simulink model "GMP_STD_CLLLC_MODEL"  (R2024b)
settings: Solver=FixedStepDiscrete  StartTime=0.0  StopTime=0.02  FixedStep=2e-8  RelTol=1e-3
PostLoadFcn:
  | gmp_model_file=get_param(bdroot,'FileName'); if isempty(gmp_model_file), error('GMP:SDPE:ModelPath','The model must be saved before SDPE initialization.'); end; gmp_model_dir=fileparts(gmp_model_file); run(fullfile(gmp_model_dir,'sdpe_mgr','ctrl_settings_matlab_init.m')); gmp_matlab_release=matlabRelease; gmp_repo_root=fullfile(gmp_model_dir,'..','..','..','..','..'); addpath(fullfile(gmp_repo_root,'slib','install_path',gmp_matlab_release.Release,'src')); clear gmp_model_file gmp_model_dir gmp_matlab_release gmp_repo_root;
InitFcn:
  | gmp_model_file=get_param(bdroot,'FileName'); if isempty(gmp_model_file), error('GMP:SDPE:ModelPath','The model must be saved before SDPE initialization.'); end; gmp_model_dir=fileparts(gmp_model_file); run(fullfile(gmp_model_dir,'sdpe_mgr','ctrl_settings_matlab_init.m')); gmp_matlab_release=matlabRelease; gmp_repo_root=fullfile(gmp_model_dir,'..','..','..','..','..'); addpath(fullfile(gmp_repo_root,'slib','install_path',gmp_matlab_release.Release,'src')); clear gmp_model_file gmp_model_dir gmp_matlab_release gmp_repo_root;
libraries: spsSeriesRLCBranchLib x4, spsCurrentMeasurementLib x3, spsUniversalBridgeLib x2, spsVoltageMeasurementLib x2, gmp_sil_core_pack x1, spsLinearTransformerLib x1, spsDCVoltageSourceLib x1, spsGroundLib x1, spspowerguiLib x1
settings Model: Creator=javnson  LastModifiedBy=javnson

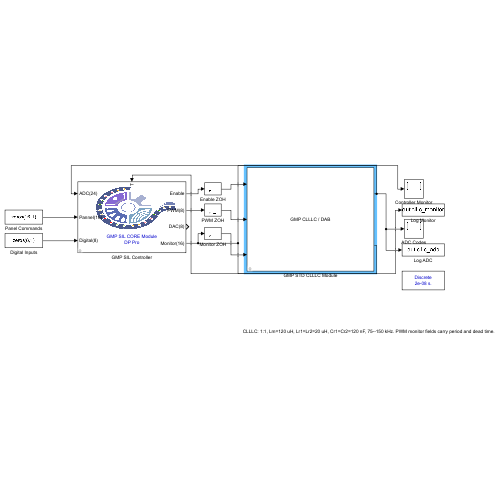
[thumbnail: Simulink's stored preview of the top-level diagram]
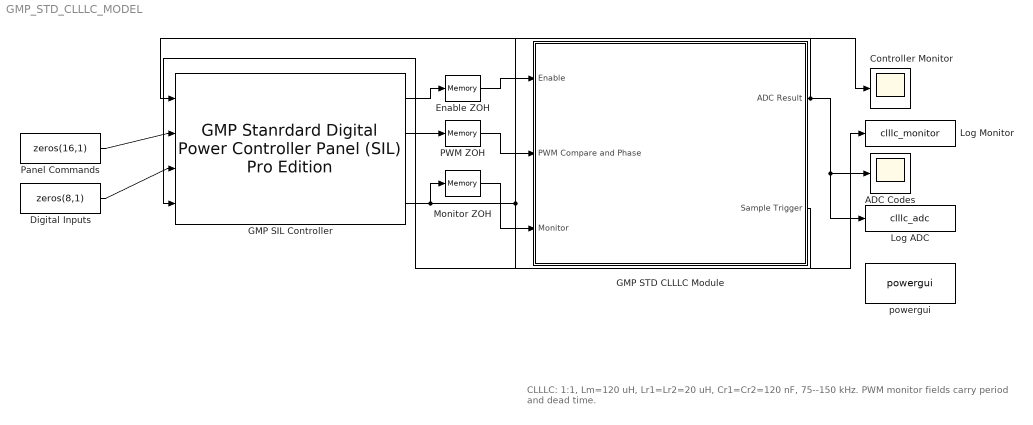
== system GMP_STD_CLLLC_MODEL ==
  note: CLLLC: 1:1, Lm=120 uH, Lr1=Lr2=20 uH, Cr1=Cr2=120 nF, 75--150 kHz. PWM monitor fields carry period and dead time.
  ADC Codes : Scope
  Controller Monitor : Scope
  Digital Inputs : Constant  Value=zeros(8,1)
  Enable ZOH : Memory
  GMP SIL Controller : gmp_sil_core_pack/GMP Stanrdard Digital Power Controller Panel (SIL) Pro Edition
      settings: SourceProductName=GMP SIL Core Utilities
  GMP STD CLLLC Module : Subsystem
      mask DialogControl TankGroup Prompt: Resonant Tank (SDPE synchronized)
      mask DialogControl SensorGroup Prompt: ADC Sensors
      mask DialogControl PwmGroup Prompt: PWM and Sampling
      mask Display: disp('GMP CLLLC / DAB')
  Log ADC : ToWorkspace  VariableName=clllc_adc  SaveFormat=Timeseries  SampleTime=-1
  Log Monitor : ToWorkspace  VariableName=clllc_monitor  SaveFormat=Timeseries  SampleTime=-1
  Monitor ZOH : Memory  InitialCondition=zeros(16,1)
  PWM ZOH : Memory  InitialCondition=zeros(8,1)
  Panel Commands : Constant  Value=zeros(16,1)
  powergui : spspowerguiLib/powergui  Priority=1  SimulationMode=Discrete  SampleTime=2e-8  frequency=60  Iterations=50  frequencyindice=60  Pbase=100e6  ErrMax=1e-4  UnitsV=kV  UnitsW=MW  buscounter=0  FunctionMessages=off  echomessages=off  EnableUseOfTLC=off  CurrentSourceSwitches=off  DisableSnubberDevices=off  DisableRonSwitches=off  DisableVfSwitches=off  DisplayEquations=off  AutomaticDiscreteSolvers=off  SolverType=Tustin/Backward Euler (TBE)  Interpol=off  ExternalGateDelay=off  methode=off  Ts=100  x0status=blocks  SPID=on  SwTol=0  HookPort=off  NonlinearTolerance=1e-4  nMaxIteration=100  ContinueOnMaxIteration=off  RestoreLinks=warning  ResistiveCurrentMeasurement=off  Frange=[0:2:500]  Ylog=off  Xlog=on  ShowGrid=off  save=off  variable=ZData  structure=0  ZoomFFT=off  StartTime=0.0  cycles=1  DisplayStyle=1  fundamental=60  FreqAxis=off  MaxFrequency=1000  frequencyindicesteady=1  RmsSteady=1  display=off
  wires:
  GMP STD CLLLC Module/1(ADC Result) -> ADC Codes/1, Log ADC/1, GMP SIL Controller/1
  Panel Commands/1 -> GMP SIL Controller/2
  Digital Inputs/1 -> GMP SIL Controller/3
  GMP STD CLLLC Module/2(Sample Trigger) -> GMP SIL Controller/4
  GMP SIL Controller/1 -> Enable ZOH/1
  GMP SIL Controller/2 -> PWM ZOH/1
  GMP SIL Controller/4 -> Controller Monitor/1, Log Monitor/1, Monitor ZOH/1
  Enable ZOH/1 -> GMP STD CLLLC Module/1(Enable)
  PWM ZOH/1 -> GMP STD CLLLC Module/2(PWM Compare and Phase)
  Monitor ZOH/1 -> GMP STD CLLLC Module/3(Monitor)

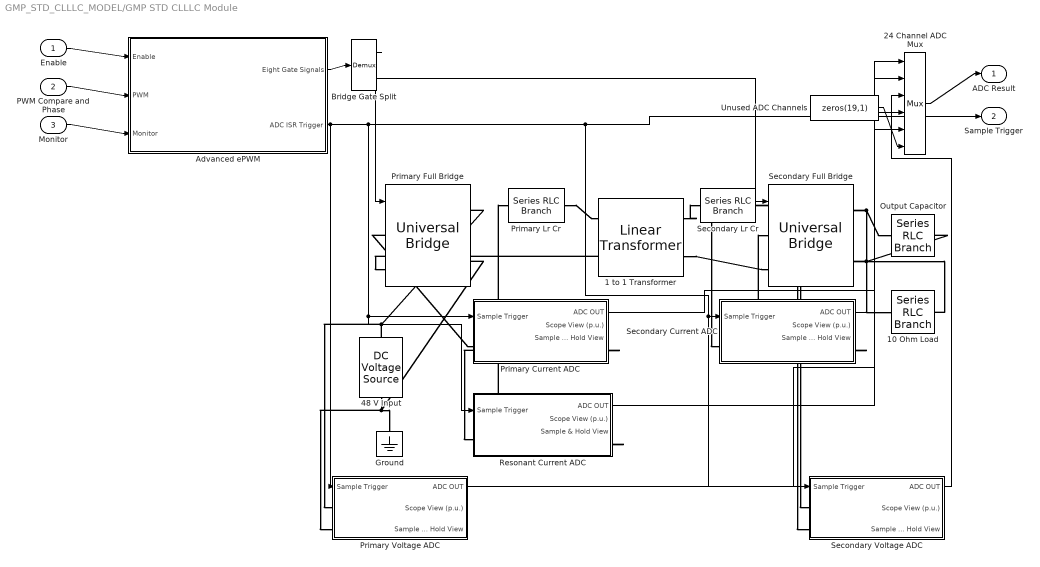
== system GMP_STD_CLLLC_MODEL/GMP STD CLLLC Module ==
  Enable : Inport
  PWM Compare and Phase : Inport  Port=2
  Monitor : Inport  Port=3
  1 to 1 Transformer : spsLinearTransformerLib/Linear Transformer  UNITS=SI  NominalPower=[1000 100e3]  winding1=[48 0.01 1e-9]  winding2=[48 0.01 1e-9]  ThreeWindings=off  winding3=[3.15e+05 0.7938 0.084225]  RmLm=[1e6 120e-6]  Measurements=None  DataType=on
  10 Ohm Load : spsSeriesRLCBranchLib/Series RLC Branch  LConnTagsString=__new0  RConnTagsString=__new0  BranchType=R  Resistance=10  Inductance=1e-3  SetiL0=off  InitialCurrent=0  Capacitance=1e-6  Setx0=off  InitialVoltage=0  Measurements=None
  24 Channel ADC Mux : Mux  Inputs=6
  48 V Input : spsDCVoltageSourceLib/DC Voltage Source  Amplitude=48  Measurements=None
  Advanced ePWM : Subsystem  mask{TimerClockHz=100e6, NominalPeriodTicks=1000, DeadtimeSeconds=200e-9, AdcCyclesPerIsr=2}
      mask prompts: TimerClockHz "Timer clock (Hz)"; NominalPeriodTicks "Nominal period ticks"; DeadtimeSeconds "Nominal dead time (s)"; AdcCyclesPerIsr "PWM cycles per ADC/ISR"
      mask DialogControl Timebase Prompt: Timebase and Frequency
      mask DialogControl Deadband Prompt: Complementary Dead Band
      mask DialogControl Sampling Prompt: ADC / ISR Trigger
      mask Display: disp('Advanced ePWM\nF/Phase/Duty/Deadtime')
  Bridge Gate Split : Demux  Outputs=[4 4]
  Ground : spsGroundLib/Ground  LConnTagsString=a
  Output Capacitor : spsSeriesRLCBranchLib/Series RLC Branch  LConnTagsString=__new0  RConnTagsString=__new0  BranchType=C  Resistance=1  Inductance=1e-3  SetiL0=off  InitialCurrent=0  Capacitance=440e-6  Setx0=off  InitialVoltage=0  Measurements=None
  Primary Current ADC : Subsystem  mask{ADC_GAIN=0.15, ADC_BIT=12, ADC_REFERENCE=3.3, ADC_BIAS=1.65, ADC_INIT=2048}
      mask DialogControl DescGroupVar Prompt: Current Sample ADC Model 1
      mask DialogControl DescTextVar Prompt: This is a ideal Current Measurement Module. This module enable a bias and a gain, and finally output a ADC result.
      mask DialogControl Control8 Prompt: ADC(p.u.) = (real_current * ADC_GAIN + ADC_BIAS)/ADC_REFERENCE
      mask DialogControl Control9 Prompt: GMP CTL Simulink Utilities: virtual peripherals
      mask DialogControl ParameterGroupVar Prompt: 参数
      mask DialogControl Control7 Prompt: ADC Current Gain (Scale Factor):
      mask DialogControl Control2 Prompt: ADC resolution:
      mask DialogControl Control4 Prompt: ADC reference Current(A), ADC full scale current (when gain = 1)
      mask DialogControl Control5 Prompt: ADC Bias Current(A)
      mask DialogControl Control6 Prompt: ADC initial Current Output(A)
  Primary Full Bridge : spsUniversalBridgeLib/Universal Bridge  Arms=2  SnubberResistance=1e6  SnubberCapacitance=inf  Device=MOSFET / Diodes  Ron=0.01  Lon=0  ForwardVoltages="[  0  0  ]"  ForwardVoltage=0  GTOparameters=[ 10e-6 , 20e-6 ]  IGBTparameters=[ 1e-6 , 2e-6 ]  Measurements=None  Measurements_2=None  converterType=Rectifier
  Primary Lr Cr : spsSeriesRLCBranchLib/Series RLC Branch  LConnTagsString=__new0  RConnTagsString=__new0  BranchType=RLC  Resistance=0.05  Inductance=20e-6  SetiL0=off  InitialCurrent=0  Capacitance=120e-9  Setx0=off  InitialVoltage=0  Measurements=None
  Primary Voltage ADC : Subsystem  mask{ADC_GAIN=0.02705, ADC_BIT=12, ADC_REFERENCE=3.3, ADC_BIAS=0, ADC_INIT=0}
      mask DialogControl DescGroupVar Prompt: Voltage Sample ADC Model
      mask DialogControl DescTextVar Prompt: This is a ideal Voltage Measurement Module.
      mask DialogControl Control2 Prompt: ADC(p.u.) = (real_voltage * ADC_GAIN + ADC_BIAS)/ADC_REFERENCE
      mask DialogControl Control9 Prompt: GMP CTL Simulink Utilities: virtual peripherals
      mask DialogControl ParameterGroupVar Prompt: Parameters:
      mask DialogControl Control4 Prompt: ADC Voltage Gain (Scale Factor):
      mask DialogControl Control5 Prompt: ADC resolution:
      mask DialogControl Control6 Prompt: ADC reference Voltage(V)
      mask DialogControl Control8 Prompt: ADC Bias Voltage(V)
      mask DialogControl Control7 Prompt: ADC Initial Voltage Output (V):
  Resonant Current ADC : Subsystem  mask{ADC_GAIN=0.15, ADC_BIT=12, ADC_REFERENCE=3.3, ADC_BIAS=1.65, ADC_INIT=2048}
      mask DialogControl DescGroupVar Prompt: Current Sample ADC Model 1
      mask DialogControl DescTextVar Prompt: This is a ideal Current Measurement Module. This module enable a bias and a gain, and finally output a ADC result.
      mask DialogControl Control8 Prompt: ADC(p.u.) = (real_current * ADC_GAIN + ADC_BIAS)/ADC_REFERENCE
      mask DialogControl Control9 Prompt: GMP CTL Simulink Utilities: virtual peripherals
      mask DialogControl ParameterGroupVar Prompt: 参数
      mask DialogControl Control7 Prompt: ADC Current Gain (Scale Factor):
      mask DialogControl Control2 Prompt: ADC resolution:
      mask DialogControl Control4 Prompt: ADC reference Current(A), ADC full scale current (when gain = 1)
      mask DialogControl Control5 Prompt: ADC Bias Current(A)
      mask DialogControl Control6 Prompt: ADC initial Current Output(A)
  Secondary Current ADC : Subsystem  mask{ADC_GAIN=0.15, ADC_BIT=12, ADC_REFERENCE=3.3, ADC_BIAS=1.65, ADC_INIT=2048}
      mask DialogControl DescGroupVar Prompt: Current Sample ADC Model 1
      mask DialogControl DescTextVar Prompt: This is a ideal Current Measurement Module. This module enable a bias and a gain, and finally output a ADC result.
      mask DialogControl Control8 Prompt: ADC(p.u.) = (real_current * ADC_GAIN + ADC_BIAS)/ADC_REFERENCE
      mask DialogControl Control9 Prompt: GMP CTL Simulink Utilities: virtual peripherals
      mask DialogControl ParameterGroupVar Prompt: 参数
      mask DialogControl Control7 Prompt: ADC Current Gain (Scale Factor):
      mask DialogControl Control2 Prompt: ADC resolution:
      mask DialogControl Control4 Prompt: ADC reference Current(A), ADC full scale current (when gain = 1)
      mask DialogControl Control5 Prompt: ADC Bias Current(A)
      mask DialogControl Control6 Prompt: ADC initial Current Output(A)
  Secondary Full Bridge : spsUniversalBridgeLib/Universal Bridge  Arms=2  SnubberResistance=1e6  SnubberCapacitance=inf  Device=MOSFET / Diodes  Ron=0.01  Lon=0  ForwardVoltages="[  0  0  ]"  ForwardVoltage=0  GTOparameters=[ 10e-6 , 20e-6 ]  IGBTparameters=[ 1e-6 , 2e-6 ]  Measurements=None  Measurements_2=None  converterType=Rectifier
  Secondary Lr Cr : spsSeriesRLCBranchLib/Series RLC Branch  LConnTagsString=__new0  RConnTagsString=__new0  BranchType=RLC  Resistance=0.05  Inductance=20e-6  SetiL0=off  InitialCurrent=0  Capacitance=120e-9  Setx0=off  InitialVoltage=0  Measurements=None
  Secondary Voltage ADC : Subsystem  mask{ADC_GAIN=0.02705, ADC_BIT=12, ADC_REFERENCE=3.3, ADC_BIAS=0, ADC_INIT=0}
      mask DialogControl DescGroupVar Prompt: Voltage Sample ADC Model
      mask DialogControl DescTextVar Prompt: This is a ideal Voltage Measurement Module.
      mask DialogControl Control2 Prompt: ADC(p.u.) = (real_voltage * ADC_GAIN + ADC_BIAS)/ADC_REFERENCE
      mask DialogControl Control9 Prompt: GMP CTL Simulink Utilities: virtual peripherals
      mask DialogControl ParameterGroupVar Prompt: Parameters:
      mask DialogControl Control4 Prompt: ADC Voltage Gain (Scale Factor):
      mask DialogControl Control5 Prompt: ADC resolution:
      mask DialogControl Control6 Prompt: ADC reference Voltage(V)
      mask DialogControl Control8 Prompt: ADC Bias Voltage(V)
      mask DialogControl Control7 Prompt: ADC Initial Voltage Output (V):
  Unused ADC Channels : Constant  Value=zeros(19,1)  OutDataTypeStr=uint32
  ADC Result : Outport
  Sample Trigger : Outport  Port=2
  wires:
  Enable/1 -> Advanced ePWM/1(Enable)
  PWM Compare and Phase/1 -> Advanced ePWM/2(PWM)
  Monitor/1 -> Advanced ePWM/3(Monitor)
  Advanced ePWM/2(ADC ISR Trigger) -> Primary Current ADC/1(Sample Trigger), Resonant Current ADC/1(Sample Trigger), Secondary Voltage ADC/1(Sample Trigger), Secondary Current ADC/1(Sample Trigger), Sample Trigger/1, Primary Voltage ADC/1(Sample Trigger)
  Advanced ePWM/1(Eight Gate Signals) -> Bridge Gate Split/1
  Bridge Gate Split/1 -> Primary Full Bridge/1
  Bridge Gate Split/2 -> Secondary Full Bridge/1
  Primary Voltage ADC/1(ADC OUT) -> 24 Channel ADC Mux/1
  Primary Current ADC/1(ADC OUT) -> 24 Channel ADC Mux/2
  Secondary Voltage ADC/1(ADC OUT) -> 24 Channel ADC Mux/3
  Secondary Current ADC/1(ADC OUT) -> 24 Channel ADC Mux/4
  Resonant Current ADC/1(ADC OUT) -> 24 Channel ADC Mux/5
  Unused ADC Channels/1 -> 24 Channel ADC Mux/6
  24 Channel ADC Mux/1 -> ADC Result/1
  connections:
  Primary Full Bridge/RConn1 -- 48 V Input/RConn1 -- Primary Voltage ADC/LConn1
  Primary Full Bridge/RConn2 -- 48 V Input/LConn1 -- Ground/LConn1 -- Primary Voltage ADC/LConn2
  Primary Full Bridge/LConn1 -- Primary Current ADC/LConn1
  Primary Current ADC/RConn1 -- Resonant Current ADC/LConn1
  Resonant Current ADC/RConn1 -- Primary Lr Cr/LConn1
  Primary Lr Cr/RConn1 -- 1 to 1 Transformer/LConn1
  1 to 1 Transformer/LConn2 -- Primary Full Bridge/LConn2
  1 to 1 Transformer/RConn1 -- Secondary Lr Cr/LConn1
  Secondary Lr Cr/RConn1 -- Secondary Current ADC/LConn1
  Secondary Current ADC/RConn1 -- Secondary Full Bridge/LConn1
  1 to 1 Transformer/RConn2 -- Secondary Full Bridge/LConn2
  Output Capacitor/LConn1 -- Secondary Full Bridge/RConn1 -- 10 Ohm Load/LConn1 -- Secondary Voltage ADC/LConn1
  Output Capacitor/RConn1 -- Secondary Full Bridge/RConn2 -- 10 Ohm Load/RConn1 -- Secondary Voltage ADC/LConn2

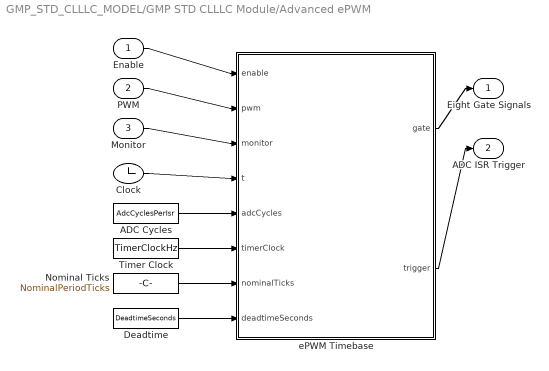
== system GMP_STD_CLLLC_MODEL/GMP STD CLLLC Module/Advanced ePWM ==
  Enable : Inport
  PWM : Inport  Port=2
  Monitor : Inport  Port=3
  ADC Cycles : Constant  Value=AdcCyclesPerIsr
  Clock : Clock
  Deadtime : Constant  Value=DeadtimeSeconds
  Nominal Ticks : Constant  Value=NominalPeriodTicks
  Timer Clock : Constant  Value=TimerClockHz
  ePWM Timebase : MATLAB Function  TreatAsAtomicUnit=on
  Eight Gate Signals : Outport
  ADC ISR Trigger : Outport  Port=2
  wires:
  Enable/1 -> ePWM Timebase/1(enable)
  PWM/1 -> ePWM Timebase/2(pwm)
  Monitor/1 -> ePWM Timebase/3(monitor)
  Clock/1 -> ePWM Timebase/4(t)
  ADC Cycles/1 -> ePWM Timebase/5(adcCycles)
  Timer Clock/1 -> ePWM Timebase/6(timerClock)
  Nominal Ticks/1 -> ePWM Timebase/7(nominalTicks)
  Deadtime/1 -> ePWM Timebase/8(deadtimeSeconds)
  ePWM Timebase/1(gate) -> Eight Gate Signals/1
  ePWM Timebase/2(trigger) -> ADC ISR Trigger/1

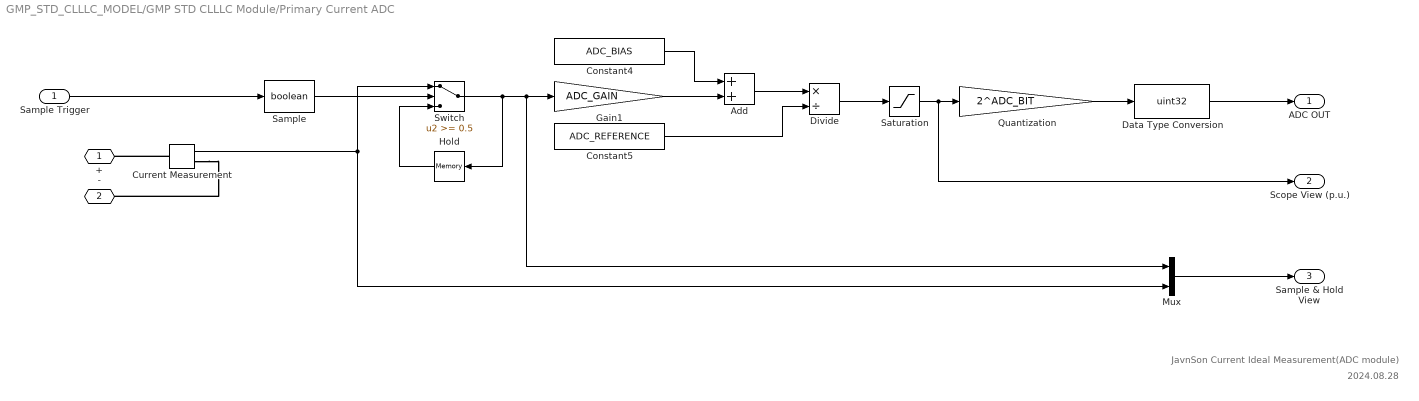
== system GMP_STD_CLLLC_MODEL/GMP STD CLLLC Module/Primary Current ADC ==
  note: 2024.08.28
  note: JavnSon Current Ideal Measurement(ADC module)
  Sample Trigger : Inport
  Add : Sum
  Constant4 : Constant  Value=ADC_BIAS
  Constant5 : Constant  Value=ADC_REFERENCE
  Current Measurement : spsCurrentMeasurementLib/Current Measurement  PhasorSimulation=off  OutputType=Complex  PSBequivalent=0
  Data Type Conversion : DataTypeConversion  OutDataTypeStr=uint32  ConvertRealWorld=Stored Integer (SI)  SaturateOnIntegerOverflow=off  RndMeth=Floor
  Divide : Product  Inputs=*/
  Gain1 : Gain  Gain=ADC_GAIN
  Hold : Memory  InitialCondition=ADC_INIT  LinearizeAsDelay=on
  Mux : Mux  Inputs=2
  Quantization : Gain  Gain=2^ADC_BIT
  Sample : DataTypeConversion  OutDataTypeStr=boolean  SaturateOnIntegerOverflow=off  RndMeth=Floor
  Saturation : Saturate  UpperLimit=1  LowerLimit=0
  Switch : Switch  Threshold=0.5
  + : PMIOPort  Side=Left
  - : PMIOPort  Port=2  Side=Right
  ADC OUT : Outport
  Scope View (p.u.) : Outport  Port=2
  Sample & Hold View : Outport  Port=3
  wires:
  Mux/1 -> Sample & Hold View/1
  Divide/1 -> Saturation/1
  Saturation/1 -> Quantization/1, Scope View (p.u.)/1
  Gain1/1 -> Add/2
  Switch/1 -> Gain1/1, Mux/1, Hold/1
  Constant4/1 -> Add/1
  Current Measurement/1 -> Switch/1, Mux/2
  Hold/1 -> Switch/3
  Data Type Conversion/1 -> ADC OUT/1
  Sample Trigger/1 -> Sample/1
  Add/1 -> Divide/1
  Sample/1 -> Switch/2
  Quantization/1 -> Data Type Conversion/1
  Constant5/1 -> Divide/2
  connections:
  Current Measurement/RConn1 -- -/RConn1
  Current Measurement/LConn1 -- +/RConn1

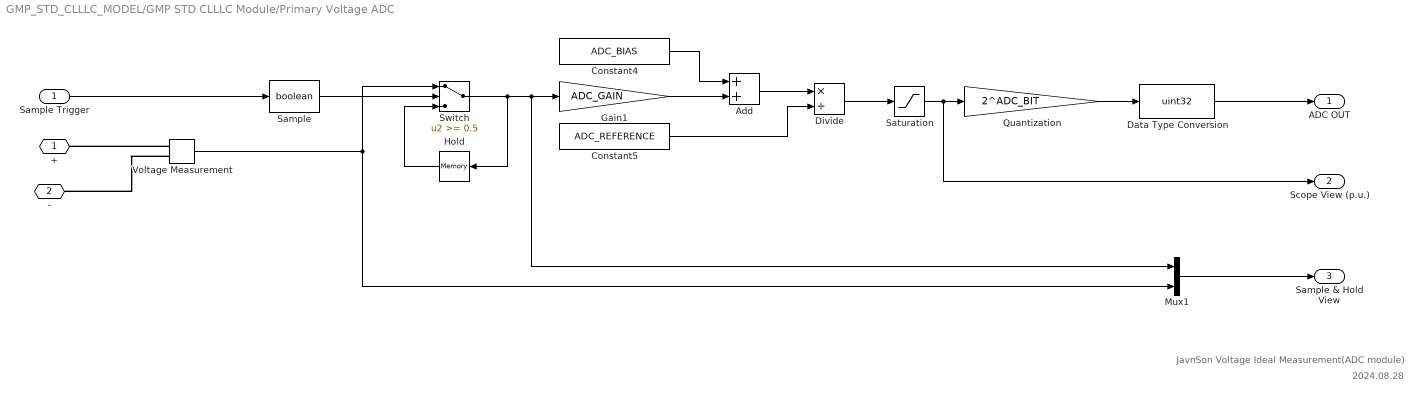
== system GMP_STD_CLLLC_MODEL/GMP STD CLLLC Module/Primary Voltage ADC ==
  note: JavnSon Voltage Ideal Measurement(ADC module)
  note: 2024.08.28
  Sample Trigger : Inport
  Add : Sum
  Constant4 : Constant  Value=ADC_BIAS
  Constant5 : Constant  Value=ADC_REFERENCE
  Data Type Conversion : DataTypeConversion  OutDataTypeStr=uint32  ConvertRealWorld=Stored Integer (SI)  SaturateOnIntegerOverflow=off  RndMeth=Floor
  Divide : Product  Inputs=*/
  Gain1 : Gain  Gain=ADC_GAIN
  Hold : Memory  InitialCondition=ADC_INIT  LinearizeAsDelay=on
  Mux1 : Mux  Inputs=2
  Quantization : Gain  Gain=2^ADC_BIT
  Sample : DataTypeConversion  OutDataTypeStr=boolean  SaturateOnIntegerOverflow=off  RndMeth=Floor
  Saturation : Saturate  UpperLimit=1  LowerLimit=0
  Switch : Switch  Threshold=0.5
  Voltage Measurement : spsVoltageMeasurementLib/Voltage Measurement  PhasorSimulation=off  OutputType=Complex  PSBequivalent=0
  + : PMIOPort  Side=Left
  - : PMIOPort  Port=2  Side=Left
  ADC OUT : Outport
  Scope View (p.u.) : Outport  Port=2
  Sample & Hold View : Outport  Port=3
  wires:
  Hold/1 -> Switch/3
  Switch/1 -> Hold/1, Mux1/1, Gain1/1
  Divide/1 -> Saturation/1
  Voltage Measurement/1 -> Mux1/2, Switch/1
  Saturation/1 -> Scope View (p.u.)/1, Quantization/1
  Constant4/1 -> Add/1
  Gain1/1 -> Add/2
  Sample Trigger/1 -> Sample/1
  Data Type Conversion/1 -> ADC OUT/1
  Mux1/1 -> Sample & Hold View/1
  Quantization/1 -> Data Type Conversion/1
  Constant5/1 -> Divide/2
  Add/1 -> Divide/1
  Sample/1 -> Switch/2
  connections:
  Voltage Measurement/LConn1 -- +/RConn1
  Voltage Measurement/LConn2 -- -/RConn1

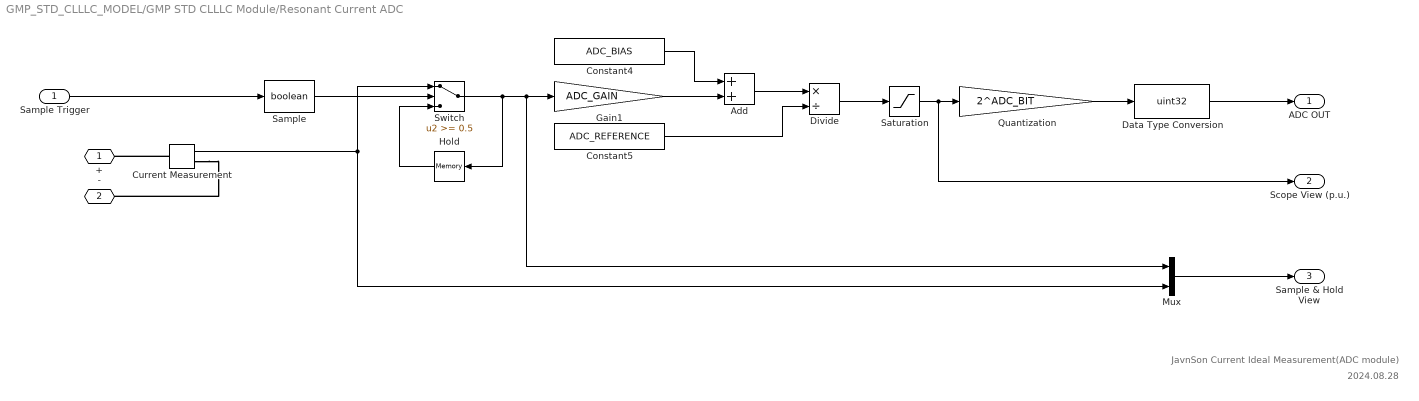
== system GMP_STD_CLLLC_MODEL/GMP STD CLLLC Module/Resonant Current ADC ==
  note: 2024.08.28
  note: JavnSon Current Ideal Measurement(ADC module)
  Sample Trigger : Inport
  Add : Sum
  Constant4 : Constant  Value=ADC_BIAS
  Constant5 : Constant  Value=ADC_REFERENCE
  Current Measurement : spsCurrentMeasurementLib/Current Measurement  PhasorSimulation=off  OutputType=Complex  PSBequivalent=0
  Data Type Conversion : DataTypeConversion  OutDataTypeStr=uint32  ConvertRealWorld=Stored Integer (SI)  SaturateOnIntegerOverflow=off  RndMeth=Floor
  Divide : Product  Inputs=*/
  Gain1 : Gain  Gain=ADC_GAIN
  Hold : Memory  InitialCondition=ADC_INIT  LinearizeAsDelay=on
  Mux : Mux  Inputs=2
  Quantization : Gain  Gain=2^ADC_BIT
  Sample : DataTypeConversion  OutDataTypeStr=boolean  SaturateOnIntegerOverflow=off  RndMeth=Floor
  Saturation : Saturate  UpperLimit=1  LowerLimit=0
  Switch : Switch  Threshold=0.5
  + : PMIOPort  Side=Left
  - : PMIOPort  Port=2  Side=Right
  ADC OUT : Outport
  Scope View (p.u.) : Outport  Port=2
  Sample & Hold View : Outport  Port=3
  wires:
  Mux/1 -> Sample & Hold View/1
  Divide/1 -> Saturation/1
  Saturation/1 -> Quantization/1, Scope View (p.u.)/1
  Gain1/1 -> Add/2
  Switch/1 -> Gain1/1, Mux/1, Hold/1
  Constant4/1 -> Add/1
  Current Measurement/1 -> Switch/1, Mux/2
  Hold/1 -> Switch/3
  Data Type Conversion/1 -> ADC OUT/1
  Sample Trigger/1 -> Sample/1
  Add/1 -> Divide/1
  Sample/1 -> Switch/2
  Quantization/1 -> Data Type Conversion/1
  Constant5/1 -> Divide/2
  connections:
  Current Measurement/RConn1 -- -/RConn1
  Current Measurement/LConn1 -- +/RConn1

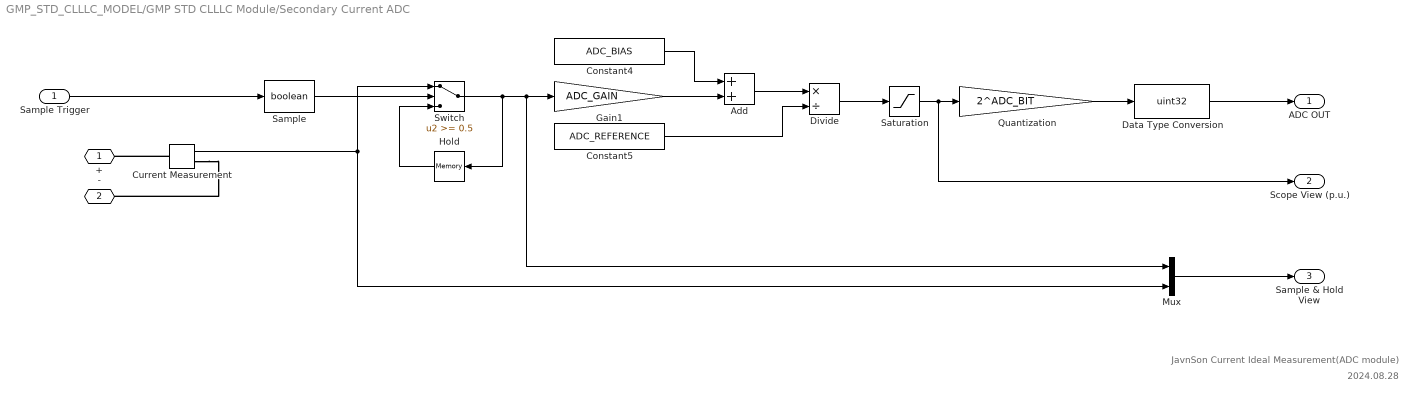
== system GMP_STD_CLLLC_MODEL/GMP STD CLLLC Module/Secondary Current ADC ==
  note: 2024.08.28
  note: JavnSon Current Ideal Measurement(ADC module)
  Sample Trigger : Inport
  Add : Sum
  Constant4 : Constant  Value=ADC_BIAS
  Constant5 : Constant  Value=ADC_REFERENCE
  Current Measurement : spsCurrentMeasurementLib/Current Measurement  PhasorSimulation=off  OutputType=Complex  PSBequivalent=0
  Data Type Conversion : DataTypeConversion  OutDataTypeStr=uint32  ConvertRealWorld=Stored Integer (SI)  SaturateOnIntegerOverflow=off  RndMeth=Floor
  Divide : Product  Inputs=*/
  Gain1 : Gain  Gain=ADC_GAIN
  Hold : Memory  InitialCondition=ADC_INIT  LinearizeAsDelay=on
  Mux : Mux  Inputs=2
  Quantization : Gain  Gain=2^ADC_BIT
  Sample : DataTypeConversion  OutDataTypeStr=boolean  SaturateOnIntegerOverflow=off  RndMeth=Floor
  Saturation : Saturate  UpperLimit=1  LowerLimit=0
  Switch : Switch  Threshold=0.5
  + : PMIOPort  Side=Left
  - : PMIOPort  Port=2  Side=Right
  ADC OUT : Outport
  Scope View (p.u.) : Outport  Port=2
  Sample & Hold View : Outport  Port=3
  wires:
  Mux/1 -> Sample & Hold View/1
  Divide/1 -> Saturation/1
  Saturation/1 -> Quantization/1, Scope View (p.u.)/1
  Gain1/1 -> Add/2
  Switch/1 -> Gain1/1, Mux/1, Hold/1
  Constant4/1 -> Add/1
  Current Measurement/1 -> Switch/1, Mux/2
  Hold/1 -> Switch/3
  Data Type Conversion/1 -> ADC OUT/1
  Sample Trigger/1 -> Sample/1
  Add/1 -> Divide/1
  Sample/1 -> Switch/2
  Quantization/1 -> Data Type Conversion/1
  Constant5/1 -> Divide/2
  connections:
  Current Measurement/RConn1 -- -/RConn1
  Current Measurement/LConn1 -- +/RConn1

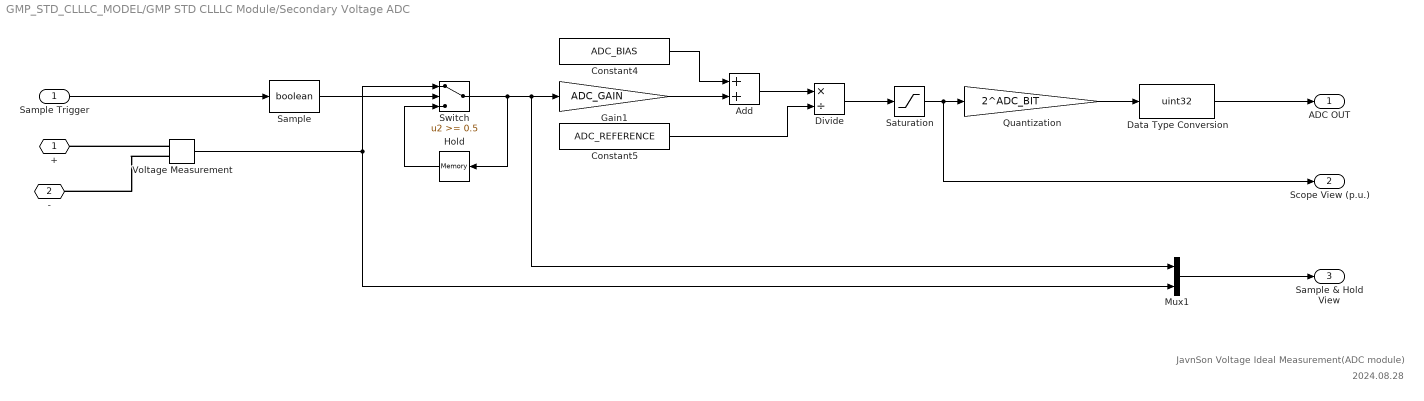
== system GMP_STD_CLLLC_MODEL/GMP STD CLLLC Module/Secondary Voltage ADC ==
  note: JavnSon Voltage Ideal Measurement(ADC module)
  note: 2024.08.28
  Sample Trigger : Inport
  Add : Sum
  Constant4 : Constant  Value=ADC_BIAS
  Constant5 : Constant  Value=ADC_REFERENCE
  Data Type Conversion : DataTypeConversion  OutDataTypeStr=uint32  ConvertRealWorld=Stored Integer (SI)  SaturateOnIntegerOverflow=off  RndMeth=Floor
  Divide : Product  Inputs=*/
  Gain1 : Gain  Gain=ADC_GAIN
  Hold : Memory  InitialCondition=ADC_INIT  LinearizeAsDelay=on
  Mux1 : Mux  Inputs=2
  Quantization : Gain  Gain=2^ADC_BIT
  Sample : DataTypeConversion  OutDataTypeStr=boolean  SaturateOnIntegerOverflow=off  RndMeth=Floor
  Saturation : Saturate  UpperLimit=1  LowerLimit=0
  Switch : Switch  Threshold=0.5
  Voltage Measurement : spsVoltageMeasurementLib/Voltage Measurement  PhasorSimulation=off  OutputType=Complex  PSBequivalent=0
  + : PMIOPort  Side=Left
  - : PMIOPort  Port=2  Side=Left
  ADC OUT : Outport
  Scope View (p.u.) : Outport  Port=2
  Sample & Hold View : Outport  Port=3
  wires:
  Hold/1 -> Switch/3
  Switch/1 -> Hold/1, Mux1/1, Gain1/1
  Divide/1 -> Saturation/1
  Voltage Measurement/1 -> Mux1/2, Switch/1
  Saturation/1 -> Scope View (p.u.)/1, Quantization/1
  Constant4/1 -> Add/1
  Gain1/1 -> Add/2
  Sample Trigger/1 -> Sample/1
  Data Type Conversion/1 -> ADC OUT/1
  Mux1/1 -> Sample & Hold View/1
  Quantization/1 -> Data Type Conversion/1
  Constant5/1 -> Divide/2
  Add/1 -> Divide/1
  Sample/1 -> Switch/2
  connections:
  Voltage Measurement/LConn1 -- +/RConn1
  Voltage Measurement/LConn2 -- -/RConn1

== matlab function GMP_STD_CLLLC_MODEL/GMP STD CLLLC Module/Advanced ePWM/ePWM Timebase ==
  data: enable input; gate output; pwm input; monitor input; t input; adcCycles input; timerClock input; nominalTicks input; deadtimeSeconds input; trigger output
function [gate,trigger] = fcn(enable,pwm,monitor,t,adcCycles,timerClock,nominalTicks,deadtimeSeconds)
% Variable-frequency, phase-shifted four-leg ePWM with complementary dead time.
persistent previous_bucket
if isempty(previous_bucket), previous_bucket = -1; end
period_pu=max(monitor(1),0.5); period=period_pu*nominalTicks/timerClock;
period_ticks=nominalTicks*period_pu; dead=max(monitor(2),deadtimeSeconds/period);
upper=false(4,1); lower=false(4,1);
for leg=1:4
 duty=min(max(double(pwm(leg))/period_ticks,0),1);
 phase=double(pwm(leg+4))/period_ticks; x=mod(t/period-phase,1);
 upper(leg)=enable>0.5 && x>=dead && x<max(duty-dead,0);
 lower(leg)=enable>0.5 && x>=min(duty+dead,1) && x<1-dead;
end
% Universal Bridge gate order is [Aupper Bupper Alower Blower].
gate=[upper(1:2);lower(1:2);upper(3:4);lower(3:4)];
bucket=floor(t/(period*max(adcCycles,1))); trigger=double(bucket~=previous_bucket); previous_bucket=bucket;
end
